simulink model "Din_Giro"  (R2020a)
settings: Solver=VariableStepAuto  StartTime=0.0  StopTime=600  RelTol=1e-3
values from neighbouring files (symbols this model uses):
  A = [-a, -b;c, -d]    [LQR_motor_cd_plot.m]    (also in Nomoto.m = [1, 0; ackerman_motor_cd_plot.m; boat.m = [a11, a12; matlab.mat = [-333.333333333  -33.3333333333; 215.754  -1.68556])
  B = [e; 0]    [LQR_motor_cd_plot.m]    (also in Nomoto.m = [y; ackerman_motor_cd_plot.m; boat.m = [b11, b12; matlab.mat = [666.666666667 0])
  C = [0, 1]    [LQR_motor_cd_plot.m]    (also in Nomoto.m = eye(2); ackerman_motor_cd_plot.m; boat.m = eye(4); matlab.mat = [0 1])
libraries: simulink x2
settings Model: Creator=micro microndas  LastModifiedBy=micro microndas

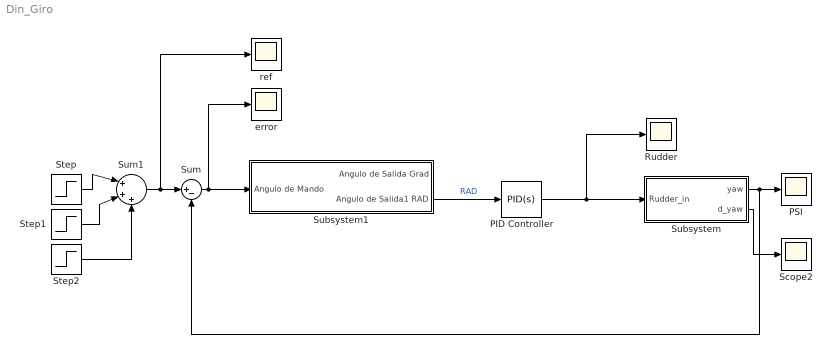
== system Din_Giro ==
  PID Controller : simulink/Continuous/PID Controller  Controller=PID  Form=Parallel  TimeDomain=Continuous-time  UseExternalTs=off  SampleTime=-1  IntegratorMethod=Forward Euler  FilterMethod=Forward Euler  ControllerParametersSource=internal  P=0.1  I=100  D=10  UseFilter=on  N=100  TunerSelectOption=Transfer Function Based (PID Tuner App)  InitialConditionSource=internal  InitialConditionForIntegrator=0  InitialConditionForFilter=0  DifferentiatorICPrevScaledInput=0  ExternalReset=none  TrackingMode=off  Kt=1  LimitOutput=off  UpperSaturationLimit=inf  LowerSaturationLimit=-inf  LinearizeAsGain=on  AntiWindupMode=none  Kb=1  POutMin=[]  POutMax=[]  IOutMin=[]  IOutMax=[]  DOutMin=[]  DOutMax=[]  NOutMin=[]  NOutMax=[]  SumOutMin=[]  SumOutMax=[]  SaturationOutMin=[]  SaturationOutMax=[]  PParamMin=[]  PParamMax=[]  IParamMin=[]  IParamMax=[]  DParamMin=[]  DParamMax=[]  NParamMin=[]  NParamMax=[]  KbParamMin=[]  KbParamMax=[]  KtParamMin=[]  KtParamMax=[]  KbOutMin=[]  KbOutMax=[]  KtOutMin=[]  KtOutMax=[]  IntegratorOutMin=[]  IntegratorOutMax=[]  FilterOutMin=[]  FilterOutMax=[]  SumI1OutMin=[]  SumI1OutMax=[]  SumI2OutMin=[]  SumI2OutMax=[]  SumI3OutMin=[]  SumI3OutMax=[]  SumI4OutMin=[]  SumI4OutMax=[]  SumDOutMin=[]  SumDOutMax=[]  DifferentiatorOutMin=[]  DifferentiatorOutMax=[]  FilterDiffOutCoefMin=[]  FilterDiffOutCoefMax=[]  ReciprocalOutMin=[]  ReciprocalOutMax=[]  SumDenOutMin=[]  SumDenOutMax=[]  SumNumOutMin=[]  SumNumOutMax=[]  DivideOutMin=[]  DivideOutMax=[]  UdiffTsProdOutMin=[]  UdiffTsProdOutMax=[]  NTsProdOutMin=[]  NTsProdOutMax=[]  UintegralTsProdOutMin=[]  UintegralTsProdOutMax=[]  UngainTsProdOutMin=[]  UngainTsProdOutMax=[]  IntegratorContinuousStateAttributes=''  IntegratorStateMustResolveToSignalObject=off  IntegratorRTWStateStorageClass=Auto  FilterContinuousStateAttributes=''  FilterStateMustResolveToSignalObject=off  FilterRTWStateStorageClass=Auto  ParallelPVariant=InternalParameters  IdealPVariant=Disabled  IVariant=InternalParameters  DVariant=InternalParameters  IntegratorVariant=Continuous  SatVariant=Disabled  AWVariant=Passthrough  PCopyVariant=Disabled  TRVariant=Disabled  FdbkBlocksVariant=Forward  IdealPFdbkVariant=Disabled  SatFdbkVariant=Disabled  DerivativeFilterVariant=ContFilter  NVariant=InternalParameters  NCopyVariant=Disabled  FilterICVariant=InternalICsFilter  IntegratorICVariant=InternalICs  ExternalResetVariant=Disabled  TRSumVariant=Passthrough  SumFdbkVariant=Disabled  SumVariant=Sum_PID  TsampFilterVariant=InternalTs  TsampNgainVariant=Passthrough  TsampIntegralVariant=Passthrough
  PSI : Scope
  Rudder : Scope
  Scope2 : Scope
  Step : Step  Time=200  Before=0.78  After=0  SampleTime=0
  Step1 : Step  Time=200  After=0.3  SampleTime=0
  Step2 : Step  Time=400  After=-0.2  SampleTime=0
  Subsystem : Subsystem
  Subsystem1 : Subsystem
  Sum : Sum  Inputs=|+-
  Sum1 : Sum  Inputs=|+++
  error : Scope
  ref : Scope
  wires:
  Step/1 -> Sum1/1
  Step1/1 -> Sum1/2
  Step2/1 -> Sum1/3
  Subsystem/1(yaw) -> Sum/2, PSI/1
  Subsystem/2(d_yaw) -> Scope2/1
  PID Controller/1 -> Rudder/1, Subsystem/1(Rudder_in)
  Subsystem1/2(Angulo de Salida1 RAD) -> PID Controller/1  "RAD"
  Sum1/1 -> ref/1, Sum/1
  Sum/1 -> error/1, Subsystem1/1(Angulo de Mando)

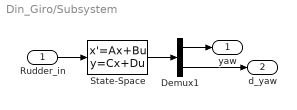
== system Din_Giro/Subsystem ==
  Rudder_in : Inport
  Demux1 : Demux  Outputs=2
  State-Space : StateSpace  A=A  B=B  C=C  D=[0;0]  InitialCondition=0  ContinuousStateAttributes={'yaw','d_yaw'}
  yaw : Outport
  d_yaw : Outport  Port=2
  wires:
  Rudder_in/1 -> State-Space/1
  State-Space/1 -> Demux1/1
  Demux1/1 -> yaw/1
  Demux1/2 -> d_yaw/1

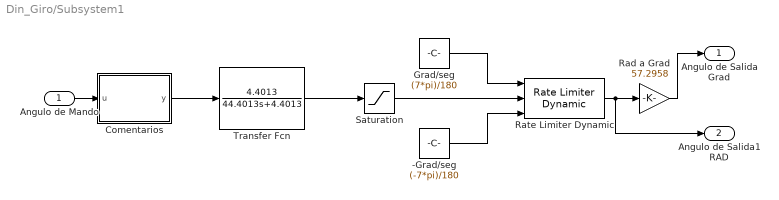
== system Din_Giro/Subsystem1 ==
  Angulo de Mando : Inport
  -Grad/seg : Constant  Value=(-7*pi)/180
  Comentarios : MATLAB Function  TreatAsAtomicUnit=on
  Grad/seg : Constant  Value=(7*pi)/180
  Rad a Grad : Gain  Gain=57.2958
  Rate Limiter Dynamic : simulink/Discontinuities/Rate Limiter Dynamic
  Saturation : Saturate  UpperLimit=pi/6  LowerLimit=-pi/6
  Transfer Fcn : TransferFcn  Numerator=[4.4013]  Denominator=[44.4013 4.4013]
  Angulo de Salida Grad : Outport
  Angulo de Salida1 RAD : Outport  Port=2
  wires:
  Grad/seg/1 -> Rate Limiter Dynamic/1
  -Grad/seg/1 -> Rate Limiter Dynamic/3
  Rate Limiter Dynamic/1 -> Angulo de Salida1 RAD/1, Rad a Grad/1
  Rad a Grad/1 -> Angulo de Salida Grad/1
  Comentarios/1(y) -> Transfer Fcn/1
  Angulo de Mando/1 -> Comentarios/1(u)
  Transfer Fcn/1 -> Saturation/1
  Saturation/1 -> Rate Limiter Dynamic/2

== matlab function Din_Giro/Subsystem1/Comentarios ==
  data: u input; y output
function y = fcn(u)

%Kg' = Kg*L / U
    %Kg = Maximo giro del timon / error maximo
        %error maximo
        %Maximo giro del timon
    %L = Eslora / Longitud del buque
        %390.00 𝑓𝑡 
        %118.872 mts
    %U = Velocidad del buque
        %15 nudo nautico
        %7.7166 m/s

y = u;
